simulink model "c00026M_harness"  (R2018a)
settings: Solver=ode3  StartTime=0.0  StopTime=10.0  RelTol=1e-3  EnableMultiTasking=on
undefined symbols (not defined in the file): b, DiscIntNeverNeededParam, J, K, L, PosMinimaW4, R, sigbuilder_block
(part 32 of 40)

== stateflow chart c00026M_harness/M008/Cyber/WL/Chart ==
  state Bajand_hasta_abajo
    entry: W = -1;
  state Bajando
    entry: W = -1;
  state Idle
    entry:W = 0;
  state Subiendo_hasta_arriba
    entry: W = 1;
  state Subiendo
    entry: W = 1;
  Subiendo -> Bajand_hasta_abajo [order 4] : [UI==4]
  Bajand_hasta_abajo -> Bajando [order 2] : [UI==3]
  Subiendo -> Bajando [order 3] : [UI==3]
  Bajando -> Bajand_hasta_abajo [order 2] : [UI==4]
  Idle -> Bajando [order 3] : [UI==3&&S>0]
  Subiendo_hasta_arriba -> Bajand_hasta_abajo [order 3] : [UI==4]
  Idle -> Bajand_hasta_abajo [order 4] : [UI==4&&S>0]
  Bajando -> Subiendo [order 3] : [UI==1]
  Subiendo_hasta_arriba -> Bajando [order 4] : [UI==3]
  Bajand_hasta_abajo -> Subiendo [order 4] : [UI==1]
  Bajand_hasta_abajo -> Idle [order 1] : [S<=0]
  Bajand_hasta_abajo -> Subiendo_hasta_arriba [order 3] : [UI==2]
  Bajando -> Idle [order 1] : [S<=0||UI==0]
  Bajando -> Subiendo_hasta_arriba [order 4] : [UI==2]
  (default) -> Idle
  Idle -> Subiendo_hasta_arriba [order 2] : [UI==2&&S<5]
  Idle -> Subiendo [order 1] : [UI == 1&&S<5]
  Subiendo -> Idle [order 1] : [S>=5||UI==0]
  Subiendo_hasta_arriba -> Idle [order 1] : [S >=5]
  Subiendo_hasta_arriba -> Subiendo [order 2] : [UI ==1]
  Subiendo -> Subiendo_hasta_arriba [order 2] : [UI==2]
  data: S input; UI input; W output double

== stateflow chart c00026M_harness/M008/Cyber/WL1/Chart1 ==
  state Bajand_hasta_abajo
    entry: W = -1;
  state Bajando
    entry: W = -1;
  state Idle
    entry:W = 0;
  state Subiendo_hasta_arriba
    entry: W = 1;
  state Subiendo
    entry: W = 1;
  Subiendo -> Bajand_hasta_abajo [order 4] : [UI==4]
  Bajand_hasta_abajo -> Bajando [order 2] : [UI==3]
  Subiendo -> Bajando [order 3] : [UI==3]
  Bajando -> Bajand_hasta_abajo [order 2] : [UI==4]
  Idle -> Bajando [order 3] : [UI==3&&S>0]
  Subiendo_hasta_arriba -> Bajand_hasta_abajo [order 3] : [UI==4]
  Idle -> Bajand_hasta_abajo [order 4] : [UI==4&&S>0]
  Bajando -> Subiendo [order 3] : [UI==1]
  Subiendo_hasta_arriba -> Bajando [order 4] : [UI==3]
  Bajand_hasta_abajo -> Subiendo [order 4] : [UI==1]
  Bajand_hasta_abajo -> Idle [order 1] : [S<=0]
  Bajand_hasta_abajo -> Subiendo_hasta_arriba [order 3] : [UI==2]
  Bajando -> Idle [order 1] : [S<=0||UI==0]
  Bajando -> Subiendo_hasta_arriba [order 4] : [UI==2]
  (default) -> Idle
  Idle -> Subiendo_hasta_arriba [order 2] : [UI==2&&S<5]
  Idle -> Subiendo [order 1] : [UI == 1&&S<5]
  Subiendo -> Idle [order 1] : [S>=5||UI==0]
  Subiendo_hasta_arriba -> Idle [order 1] : [S >=5]
  Subiendo_hasta_arriba -> Subiendo [order 2] : [UI ==1]
  Subiendo -> Subiendo_hasta_arriba [order 2] : [UI==2]
  data: S input; UI input; W output double

== stateflow chart c00026M_harness/M008/Cyber/WL3/Chart2 ==
  state Bajand_hasta_abajo
    entry: W = -1;
  state Bajando
    entry: W = -1;
  state Idle
    entry:W = 0;
  state Subiendo_hasta_arriba
    entry: W = 1;
  state Subiendo
    entry: W = 1;
  Subiendo -> Bajand_hasta_abajo [order 4] : [UI==4]
  Bajand_hasta_abajo -> Bajando [order 2] : [UI==3]
  Subiendo -> Bajando [order 3] : [UI==3]
  Bajando -> Bajand_hasta_abajo [order 2] : [UI==4]
  Idle -> Bajando [order 3] : [UI==3&&S>PosMinW4]
  Subiendo_hasta_arriba -> Bajand_hasta_abajo [order 3] : [UI==4]
  Idle -> Bajand_hasta_abajo [order 4] : [UI==4&&S>PosMinW4]
  Bajando -> Subiendo [order 3] : [UI==1]
  Subiendo_hasta_arriba -> Bajando [order 4] : [UI==3]
  Bajand_hasta_abajo -> Subiendo [order 4] : [UI==1]
  Bajand_hasta_abajo -> Idle [order 1] : [S<=PosMinW4]
  Bajand_hasta_abajo -> Subiendo_hasta_arriba [order 3] : [UI==2]
  Bajando -> Idle [order 1] : [S<=PosMinW4||UI==0]
  Bajando -> Subiendo_hasta_arriba [order 4] : [UI==2]
  (default) -> Idle
  Idle -> Subiendo_hasta_arriba [order 2] : [UI==2&&S<5]
  Idle -> Subiendo [order 1] : [UI == 1&&S<5]
  Subiendo -> Idle [order 1] : [S>=5||UI==0]
  Subiendo_hasta_arriba -> Idle [order 1] : [S >=5]
  Subiendo_hasta_arriba -> Subiendo [order 2] : [UI ==1]
  Subiendo -> Subiendo_hasta_arriba [order 2] : [UI==2]
  data: S input; UI input; W output double; PosMinW4 input

== stateflow chart c00026M_harness/M009/Cyber/WL/Chart ==
  state Bajand_hasta_abajo
    entry: W = -1;
  state Bajando
    entry: W = -1;
  state Idle
    entry:W = 0;
  state Subiendo_hasta_arriba
    entry: W = 1;
  state Subiendo
    entry: W = 1;
  Subiendo -> Bajand_hasta_abajo [order 4] : [UI==4]
  Bajand_hasta_abajo -> Bajando [order 2] : [UI==3]
  Subiendo -> Bajando [order 3] : [UI==3]
  Bajando -> Bajand_hasta_abajo [order 2] : [UI==4]
  Idle -> Bajando [order 3] : [UI==3&&S>0]
  Subiendo_hasta_arriba -> Bajand_hasta_abajo [order 3] : [UI==4]
  Idle -> Bajand_hasta_abajo [order 4] : [UI==4&&S>0]
  Bajando -> Subiendo [order 3] : [UI==1]
  Subiendo_hasta_arriba -> Bajando [order 4] : [UI==3]
  Bajand_hasta_abajo -> Subiendo [order 4] : [UI==1]
  Bajand_hasta_abajo -> Idle [order 1] : [S<=0]
  Bajand_hasta_abajo -> Subiendo_hasta_arriba [order 3] : [UI==2]
  Bajando -> Idle [order 1] : [S<=0||UI==0]
  Bajando -> Subiendo_hasta_arriba [order 4] : [UI==2]
  (default) -> Idle
  Idle -> Subiendo_hasta_arriba [order 2] : [UI==2&&S<5]
  Idle -> Subiendo [order 1] : [UI == 1&&S<5]
  Subiendo -> Idle [order 1] : [S>=5||UI==0]
  Subiendo_hasta_arriba -> Idle [order 1] : [S >=5]
  Subiendo_hasta_arriba -> Subiendo [order 2] : [UI ==1]
  Subiendo -> Subiendo_hasta_arriba [order 2] : [UI==2]
  data: S input; UI input; W output double

== stateflow chart c00026M_harness/M009/Cyber/WL1/Chart1 ==
  state Bajand_hasta_abajo
    entry: W = -1;
  state Bajando
    entry: W = -1;
  state Idle
    entry:W = 0;
  state Subiendo_hasta_arriba
    entry: W = 1;
  state Subiendo
    entry: W = 1;
  Subiendo -> Bajand_hasta_abajo [order 4] : [UI==4]
  Bajand_hasta_abajo -> Bajando [order 2] : [UI==3]
  Subiendo -> Bajando [order 3] : [UI==3]
  Bajando -> Bajand_hasta_abajo [order 2] : [UI==4]
  Idle -> Bajando [order 3] : [UI==3&&S>0]
  Subiendo_hasta_arriba -> Bajand_hasta_abajo [order 3] : [UI==4]
  Idle -> Bajand_hasta_abajo [order 4] : [UI==4&&S>0]
  Bajando -> Subiendo [order 3] : [UI==1]
  Subiendo_hasta_arriba -> Bajando [order 4] : [UI==3]
  Bajand_hasta_abajo -> Subiendo [order 4] : [UI==1]
  Bajand_hasta_abajo -> Idle [order 1] : [S<=0]
  Bajand_hasta_abajo -> Subiendo_hasta_arriba [order 3] : [UI==2]
  Bajando -> Idle [order 1] : [S<=0||UI==0]
  Bajando -> Subiendo_hasta_arriba [order 4] : [UI==2]
  (default) -> Idle
  Idle -> Subiendo_hasta_arriba [order 2] : [UI==2&&S<5]
  Idle -> Subiendo [order 1] : [UI == 1&&S<5]
  Subiendo -> Idle [order 1] : [S>=5||UI==0]
  Subiendo_hasta_arriba -> Idle [order 1] : [S >=5]
  Subiendo_hasta_arriba -> Subiendo [order 2] : [UI ==1]
  Subiendo -> Subiendo_hasta_arriba [order 2] : [UI==2]
  data: S input; UI input; W output double

== stateflow chart c00026M_harness/M009/Cyber/WL3/Chart2 ==
  state Bajand_hasta_abajo
    entry: W = -1;
  state Bajando
    entry: W = -1;
  state Idle
    entry:W = 0;
  state Subiendo_hasta_arriba
    entry: W = 1;
  state Subiendo
    entry: W = 1;
  Subiendo -> Bajand_hasta_abajo [order 4] : [UI==4]
  Bajand_hasta_abajo -> Bajando [order 2] : [UI==3]
  Subiendo -> Bajando [order 3] : [UI==3]
  Bajando -> Bajand_hasta_abajo [order 2] : [UI==4]
  Idle -> Bajando [order 3] : [UI==3&&S>PosMinW4]
  Subiendo_hasta_arriba -> Bajand_hasta_abajo [order 3] : [UI==4]
  Idle -> Bajand_hasta_abajo [order 4] : [UI==4&&S>PosMinW4]
  Bajando -> Subiendo [order 3] : [UI==1]
  Subiendo_hasta_arriba -> Bajando [order 4] : [UI==3]
  Bajand_hasta_abajo -> Subiendo [order 4] : [UI==1]
  Bajand_hasta_abajo -> Idle [order 1] : [S<=PosMinW4]
  Bajand_hasta_abajo -> Subiendo_hasta_arriba [order 3] : [UI==2]
  Bajando -> Idle [order 1] : [S<=PosMinW4||UI==0]
  Bajando -> Subiendo_hasta_arriba [order 4] : [UI==2]
  (default) -> Idle
  Idle -> Subiendo_hasta_arriba [order 2] : [UI==2&&S<5]
  Idle -> Subiendo [order 1] : [UI == 1&&S<5]
  Subiendo -> Idle [order 1] : [S>=5||UI==0]
  Subiendo_hasta_arriba -> Idle [order 1] : [S >=5]
  Subiendo_hasta_arriba -> Subiendo [order 2] : [UI ==1]
  Subiendo -> Subiendo_hasta_arriba [order 2] : [UI==2]
  data: S input; UI input; W output double; PosMinW4 input

== stateflow chart c00026M_harness/M010/Cyber/WL/Chart ==
  state Bajand_hasta_abajo
    entry: W = -1;
  state Bajando
    entry: W = -1;
  state Idle
    entry:W = 0;
  state Subiendo_hasta_arriba
    entry: W = 1;
  state Subiendo
    entry: W = 1;
  Subiendo -> Bajand_hasta_abajo [order 4] : [UI==4]
  Bajand_hasta_abajo -> Bajando [order 2] : [UI==3]
  Subiendo -> Bajando [order 3] : [UI==3]
  Bajando -> Bajand_hasta_abajo [order 2] : [UI==4]
  Idle -> Bajando [order 3] : [UI==3&&S>0]
  Subiendo_hasta_arriba -> Bajand_hasta_abajo [order 3] : [UI==4]
  Idle -> Bajand_hasta_abajo [order 4] : [UI==4&&S>0]
  Bajando -> Subiendo [order 3] : [UI==1]
  Subiendo_hasta_arriba -> Bajando [order 4] : [UI==3]
  Bajand_hasta_abajo -> Subiendo [order 4] : [UI==1]
  Bajand_hasta_abajo -> Idle [order 1] : [S<=0]
  Bajand_hasta_abajo -> Subiendo_hasta_arriba [order 3] : [UI==2]
  Bajando -> Idle [order 1] : [S<=0||UI==0]
  Bajando -> Subiendo_hasta_arriba [order 4] : [UI==2]
  (default) -> Idle
  Idle -> Subiendo_hasta_arriba [order 2] : [UI==2&&S<5]
  Idle -> Subiendo [order 1] : [UI == 1&&S<5]
  Subiendo -> Idle [order 1] : [S>=5||UI==0]
  Subiendo_hasta_arriba -> Idle [order 1] : [S >=5]
  Subiendo_hasta_arriba -> Subiendo [order 2] : [UI ==1]
  Subiendo -> Subiendo_hasta_arriba [order 2] : [UI==2]
  data: S input; UI input; W output double

== stateflow chart c00026M_harness/M010/Cyber/WL1/Chart1 ==
  state Bajand_hasta_abajo
    entry: W = -1;
  state Bajando
    entry: W = -1;
  state Idle
    entry:W = 0;
  state Subiendo_hasta_arriba
    entry: W = 1;
  state Subiendo
    entry: W = 1;
  Subiendo -> Bajand_hasta_abajo [order 4] : [UI==4]
  Bajand_hasta_abajo -> Bajando [order 2] : [UI==3]
  Subiendo -> Bajando [order 3] : [UI==3]
  Bajando -> Bajand_hasta_abajo [order 2] : [UI==4]
  Idle -> Bajando [order 3] : [UI==3&&S>0]
  Subiendo_hasta_arriba -> Bajand_hasta_abajo [order 3] : [UI==4]
  Idle -> Bajand_hasta_abajo [order 4] : [UI==4&&S>0]
  Bajando -> Subiendo [order 3] : [UI==1]
  Subiendo_hasta_arriba -> Bajando [order 4] : [UI==3]
  Bajand_hasta_abajo -> Subiendo [order 4] : [UI==1]
  Bajand_hasta_abajo -> Idle [order 1] : [S<=0]
  Bajand_hasta_abajo -> Subiendo_hasta_arriba [order 3] : [UI==2]
  Bajando -> Idle [order 1] : [S<=0||UI==0]
  Bajando -> Subiendo_hasta_arriba [order 4] : [UI==2]
  (default) -> Idle
  Idle -> Subiendo_hasta_arriba [order 2] : [UI==2&&S<5]
  Idle -> Subiendo [order 1] : [UI == 1&&S<5]
  Subiendo -> Idle [order 1] : [S>=5||UI==0]
  Subiendo_hasta_arriba -> Idle [order 1] : [S >=5]
  Subiendo_hasta_arriba -> Subiendo [order 2] : [UI ==1]
  Subiendo -> Subiendo_hasta_arriba [order 2] : [UI==2]
  data: S input; UI input; W output double

== stateflow chart c00026M_harness/M010/Cyber/WL3/Chart2 ==
  state Bajand_hasta_abajo
    entry: W = -1;
  state Bajando
    entry: W = -1;
  state Idle
    entry:W = 0;
  state Subiendo_hasta_arriba
    entry: W = 1;
  state Subiendo
    entry: W = 1;
  Subiendo -> Bajand_hasta_abajo [order 4] : [UI==4]
  Bajand_hasta_abajo -> Bajando [order 2] : [UI==3]
  Subiendo -> Bajando [order 3] : [UI==3]
  Bajando -> Bajand_hasta_abajo [order 2] : [UI==4]
  Idle -> Bajando [order 3] : [UI==3&&S>PosMinW4]
  Subiendo_hasta_arriba -> Bajand_hasta_abajo [order 3] : [UI==4]
  Idle -> Bajand_hasta_abajo [order 4] : [UI==4&&S>PosMinW4]
  Bajando -> Subiendo [order 3] : [UI==1]
  Subiendo_hasta_arriba -> Bajando [order 4] : [UI==3]
  Bajand_hasta_abajo -> Subiendo [order 4] : [UI==1]
  Bajand_hasta_abajo -> Idle [order 1] : [S<=PosMinW4]
  Bajand_hasta_abajo -> Subiendo_hasta_arriba [order 3] : [UI==2]
  Bajando -> Idle [order 1] : [S<=PosMinW4||UI==0]
  Bajando -> Subiendo_hasta_arriba [order 4] : [UI==2]
  (default) -> Idle
  Idle -> Subiendo_hasta_arriba [order 2] : [UI==2&&S<5]
  Idle -> Subiendo [order 1] : [UI == 1&&S<5]
  Subiendo -> Idle [order 1] : [S>=5||UI==0]
  Subiendo_hasta_arriba -> Idle [order 1] : [S >=5]
  Subiendo_hasta_arriba -> Subiendo [order 2] : [UI ==1]
  Subiendo -> Subiendo_hasta_arriba [order 2] : [UI==2]
  data: S input; UI input; W output double; PosMinW4 input

== stateflow chart c00026M_harness/M011/Cyber/WL/Chart ==
  state Bajand_hasta_abajo
    entry: W = -1;
  state Bajando
    entry: W = -1;
  state Idle
    entry:W = 0;
  state Subiendo_hasta_arriba
    entry: W = 1;
  state Subiendo
    entry: W = 1;
  Subiendo -> Bajand_hasta_abajo [order 4] : [UI==4]
  Bajand_hasta_abajo -> Bajando [order 2] : [UI==3]
  Subiendo -> Bajando [order 3] : [UI==3]
  Bajando -> Bajand_hasta_abajo [order 2] : [UI==4]
  Idle -> Bajando [order 3] : [UI==3&&S>0]
  Subiendo_hasta_arriba -> Bajand_hasta_abajo [order 3] : [UI==4]
  Idle -> Bajand_hasta_abajo [order 4] : [UI==4&&S>0]
  Bajando -> Subiendo [order 3] : [UI==1]
  Subiendo_hasta_arriba -> Bajando [order 4] : [UI==3]
  Bajand_hasta_abajo -> Subiendo [order 4] : [UI==1]
  Bajand_hasta_abajo -> Idle [order 1] : [S<=0]
  Bajand_hasta_abajo -> Subiendo_hasta_arriba [order 3] : [UI==2]
  Bajando -> Idle [order 1] : [S<=0||UI==0]
  Bajando -> Subiendo_hasta_arriba [order 4] : [UI==2]
  (default) -> Idle
  Idle -> Subiendo_hasta_arriba [order 2] : [UI==2&&S<5]
  Idle -> Subiendo [order 1] : [UI == 1&&S<5]
  Subiendo -> Idle [order 1] : [S>=5||UI==0]
  Subiendo_hasta_arriba -> Idle [order 1] : [S >=5]
  Subiendo_hasta_arriba -> Subiendo [order 2] : [UI ==1]
  Subiendo -> Subiendo_hasta_arriba [order 2] : [UI==2]
  data: S input; UI input; W output double

== stateflow chart c00026M_harness/M011/Cyber/WL1/Chart1 ==
  state Bajand_hasta_abajo
    entry: W = -1;
  state Bajando
    entry: W = -1;
  state Idle
    entry:W = 0;
  state Subiendo_hasta_arriba
    entry: W = 1;
  state Subiendo
    entry: W = 1;
  Subiendo -> Bajand_hasta_abajo [order 4] : [UI==4]
  Bajand_hasta_abajo -> Bajando [order 2] : [UI==3]
  Subiendo -> Bajando [order 3] : [UI==3]
  Bajando -> Bajand_hasta_abajo [order 2] : [UI==4]
  Idle -> Bajando [order 3] : [UI==3&&S>0]
  Subiendo_hasta_arriba -> Bajand_hasta_abajo [order 3] : [UI==4]
  Idle -> Bajand_hasta_abajo [order 4] : [UI==4&&S>0]
  Bajando -> Subiendo [order 3] : [UI==1]
  Subiendo_hasta_arriba -> Bajando [order 4] : [UI==3]
  Bajand_hasta_abajo -> Subiendo [order 4] : [UI==1]
  Bajand_hasta_abajo -> Idle [order 1] : [S<=0]
  Bajand_hasta_abajo -> Subiendo_hasta_arriba [order 3] : [UI==2]
  Bajando -> Idle [order 1] : [S<=0||UI==0]
  Bajando -> Subiendo_hasta_arriba [order 4] : [UI==2]
  (default) -> Idle
  Idle -> Subiendo_hasta_arriba [order 2] : [UI==2&&S<5]
  Idle -> Subiendo [order 1] : [UI == 1&&S<5]
  Subiendo -> Idle [order 1] : [S>=5||UI==0]
  Subiendo_hasta_arriba -> Idle [order 1] : [S >=5]
  Subiendo_hasta_arriba -> Subiendo [order 2] : [UI ==1]
  Subiendo -> Subiendo_hasta_arriba [order 2] : [UI==2]
  data: S input; UI input; W output double

== stateflow chart c00026M_harness/M011/Cyber/WL3/Chart2 ==
  state Bajand_hasta_abajo
    entry: W = -1;
  state Bajando
    entry: W = -1;
  state Idle
    entry:W = 0;
  state Subiendo_hasta_arriba
    entry: W = 1;
  state Subiendo
    entry: W = 1;
  Subiendo -> Bajand_hasta_abajo [order 4] : [UI==4]
  Bajand_hasta_abajo -> Bajando [order 2] : [UI==3]
  Subiendo -> Bajando [order 3] : [UI==3]
  Bajando -> Bajand_hasta_abajo [order 2] : [UI==4]
  Idle -> Bajando [order 3] : [UI==3&&S>PosMinW4]
  Subiendo_hasta_arriba -> Bajand_hasta_abajo [order 3] : [UI==4]
  Idle -> Bajand_hasta_abajo [order 4] : [UI==4&&S>PosMinW4]
  Bajando -> Subiendo [order 3] : [UI==1]
  Subiendo_hasta_arriba -> Bajando [order 4] : [UI==3]
  Bajand_hasta_abajo -> Subiendo [order 4] : [UI==1]
  Bajand_hasta_abajo -> Idle [order 1] : [S<=PosMinW4]
  Bajand_hasta_abajo -> Subiendo_hasta_arriba [order 3] : [UI==2]
  Bajando -> Idle [order 1] : [S<=PosMinW4||UI==0]
  Bajando -> Subiendo_hasta_arriba [order 4] : [UI==2]
  (default) -> Idle
  Idle -> Subiendo_hasta_arriba [order 2] : [UI==2&&S<5]
  Idle -> Subiendo [order 1] : [UI == 1&&S<5]
  Subiendo -> Idle [order 1] : [S>=5||UI==0]
  Subiendo_hasta_arriba -> Idle [order 1] : [S >=5]
  Subiendo_hasta_arriba -> Subiendo [order 2] : [UI ==1]
  Subiendo -> Subiendo_hasta_arriba [order 2] : [UI==2]
  data: S input; UI input; W output double; PosMinW4 input

== stateflow chart c00026M_harness/M012/Cyber/WL/Chart ==
  state Bajand_hasta_abajo
    entry: W = -1;
  state Bajando
    entry: W = -1;
  state Idle
    entry:W = 0;
  state Subiendo_hasta_arriba
    entry: W = 1;
  state Subiendo
    entry: W = 1;
  Subiendo -> Bajand_hasta_abajo [order 4] : [UI==4]
  Bajand_hasta_abajo -> Bajando [order 2] : [UI==3]
  Subiendo -> Bajando [order 3] : [UI==3]
  Bajando -> Bajand_hasta_abajo [order 2] : [UI==4]
  Idle -> Bajando [order 3] : [UI==3&&S>0]
  Subiendo_hasta_arriba -> Bajand_hasta_abajo [order 3] : [UI==4]
  Idle -> Bajand_hasta_abajo [order 4] : [UI==4&&S>0]
  Bajando -> Subiendo [order 3] : [UI==1]
  Subiendo_hasta_arriba -> Bajando [order 4] : [UI==3]
  Bajand_hasta_abajo -> Subiendo [order 4] : [UI==1]
  Bajand_hasta_abajo -> Idle [order 1] : [S<=0]
  Bajand_hasta_abajo -> Subiendo_hasta_arriba [order 3] : [UI==2]
  Bajando -> Idle [order 1] : [S<=0||UI==0]
  Bajando -> Subiendo_hasta_arriba [order 4] : [UI==2]
  (default) -> Idle
  Idle -> Subiendo_hasta_arriba [order 2] : [UI==2&&S<5]
  Idle -> Subiendo [order 1] : [UI == 1&&S<5]
  Subiendo -> Idle [order 1] : [S>=5||UI==0]
  Subiendo_hasta_arriba -> Idle [order 1] : [S >=5]
  Subiendo_hasta_arriba -> Subiendo [order 2] : [UI ==1]
  Subiendo -> Subiendo_hasta_arriba [order 2] : [UI==2]
  data: S input; UI input; W output double

== stateflow chart c00026M_harness/M012/Cyber/WL1/Chart1 ==
  state Bajand_hasta_abajo
    entry: W = -1;
  state Bajando
    entry: W = -1;
  state Idle
    entry:W = 0;
  state Subiendo_hasta_arriba
    entry: W = 1;
  state Subiendo
    entry: W = 1;
  Subiendo -> Bajand_hasta_abajo [order 4] : [UI==4]
  Bajand_hasta_abajo -> Bajando [order 2] : [UI==3]
  Subiendo -> Bajando [order 3] : [UI==3]
  Bajando -> Bajand_hasta_abajo [order 2] : [UI==4]
  Idle -> Bajando [order 3] : [UI==3&&S>0]
  Subiendo_hasta_arriba -> Bajand_hasta_abajo [order 3] : [UI==4]
  Idle -> Bajand_hasta_abajo [order 4] : [UI==4&&S>0]
  Bajando -> Subiendo [order 3] : [UI==1]
  Subiendo_hasta_arriba -> Bajando [order 4] : [UI==3]
  Bajand_hasta_abajo -> Subiendo [order 4] : [UI==1]
  Bajand_hasta_abajo -> Idle [order 1] : [S<=0]
  Bajand_hasta_abajo -> Subiendo_hasta_arriba [order 3] : [UI==2]
  Bajando -> Idle [order 1] : [S<=0||UI==0]
  Bajando -> Subiendo_hasta_arriba [order 4] : [UI==2]
  (default) -> Idle
  Idle -> Subiendo_hasta_arriba [order 2] : [UI==2&&S<5]
  Idle -> Subiendo [order 1] : [UI == 1&&S<5]
  Subiendo -> Idle [order 1] : [S>=5||UI==0]
  Subiendo_hasta_arriba -> Idle [order 1] : [S >=5]
  Subiendo_hasta_arriba -> Subiendo [order 2] : [UI ==1]
  Subiendo -> Subiendo_hasta_arriba [order 2] : [UI==2]
  data: S input; UI input; W output double

== stateflow chart c00026M_harness/M012/Cyber/WL3/Chart2 ==
  state Bajand_hasta_abajo
    entry: W = -1;
  state Bajando
    entry: W = -1;
  state Idle
    entry:W = 0;
  state Subiendo_hasta_arriba
    entry: W = 1;
  state Subiendo
    entry: W = 1;
  Subiendo -> Bajand_hasta_abajo [order 4] : [UI==4]
  Bajand_hasta_abajo -> Bajando [order 2] : [UI==3]
  Subiendo -> Bajando [order 3] : [UI==3]
  Bajando -> Bajand_hasta_abajo [order 2] : [UI==4]
  Idle -> Bajando [order 3] : [UI==3&&S>PosMinW4]
  Subiendo_hasta_arriba -> Bajand_hasta_abajo [order 3] : [UI==4]
  Idle -> Bajand_hasta_abajo [order 4] : [UI==4&&S>PosMinW4]
  Bajando -> Subiendo [order 3] : [UI==1]
  Subiendo_hasta_arriba -> Bajando [order 4] : [UI==3]
  Bajand_hasta_abajo -> Subiendo [order 4] : [UI==1]
  Bajand_hasta_abajo -> Idle [order 1] : [S<=PosMinW4]
  Bajand_hasta_abajo -> Subiendo_hasta_arriba [order 3] : [UI==2]
  Bajando -> Idle [order 1] : [S<=PosMinW4||UI==0]
  Bajando -> Subiendo_hasta_arriba [order 4] : [UI==2]
  (default) -> Idle
  Idle -> Subiendo_hasta_arriba [order 2] : [UI==2&&S<5]
  Idle -> Subiendo [order 1] : [UI == 1&&S<5]
  Subiendo -> Idle [order 1] : [S>=5||UI==0]
  Subiendo_hasta_arriba -> Idle [order 1] : [S >=5]
  Subiendo_hasta_arriba -> Subiendo [order 2] : [UI ==1]
  Subiendo -> Subiendo_hasta_arriba [order 2] : [UI==2]
  data: S input; UI input; W output double; PosMinW4 input

== stateflow chart c00026M_harness/M014/Cyber/WL/Chart ==
  state Bajand_hasta_abajo
    entry: W = -1;
  state Bajando
    entry: W = -1;
  state Idle
    entry:W = 0;
  state Subiendo_hasta_arriba
    entry: W = 1;
  state Subiendo
    entry: W = 1;
  Subiendo -> Bajand_hasta_abajo [order 4] : [UI==4]
  Bajand_hasta_abajo -> Bajando [order 2] : [UI==3]
  Subiendo -> Bajando [order 3] : [UI==3]
  Bajando -> Bajand_hasta_abajo [order 2] : [UI==4]
  Idle -> Bajando [order 3] : [UI==3&&S>0]
  Subiendo_hasta_arriba -> Bajand_hasta_abajo [order 3] : [UI==4]
  Idle -> Bajand_hasta_abajo [order 4] : [UI==4&&S>0]
  Bajando -> Subiendo [order 3] : [UI==1]
  Subiendo_hasta_arriba -> Bajando [order 4] : [UI==3]
  Bajand_hasta_abajo -> Subiendo [order 4] : [UI==1]
  Bajand_hasta_abajo -> Idle [order 1] : [S<=0]
  Bajand_hasta_abajo -> Subiendo_hasta_arriba [order 3] : [UI==2]
  Bajando -> Idle [order 1] : [S<=0||UI==0]
  Bajando -> Subiendo_hasta_arriba [order 4] : [UI==2]
  (default) -> Idle
  Idle -> Subiendo_hasta_arriba [order 2] : [UI==2&&S<5]
  Idle -> Subiendo [order 1] : [UI == 1&&S<5]
  Subiendo -> Idle [order 1] : [S>=5||UI==0]
  Subiendo_hasta_arriba -> Idle [order 1] : [S >=5]
  Subiendo_hasta_arriba -> Subiendo [order 2] : [UI ==1]
  Subiendo -> Subiendo_hasta_arriba [order 2] : [UI==2]
  data: S input; UI input; W output double

== stateflow chart c00026M_harness/M014/Cyber/WL1/Chart1 ==
  state Bajand_hasta_abajo
    entry: W = -1;
  state Bajando
    entry: W = -1;
  state Idle
    entry:W = 0;
  state Subiendo_hasta_arriba
    entry: W = 1;
  state Subiendo
    entry: W = 1;
  Subiendo -> Bajand_hasta_abajo [order 4] : [UI==4]
  Bajand_hasta_abajo -> Bajando [order 2] : [UI==3]
  Subiendo -> Bajando [order 3] : [UI==3]
  Bajando -> Bajand_hasta_abajo [order 2] : [UI==4]
  Idle -> Bajando [order 3] : [UI==3&&S>0]
  Subiendo_hasta_arriba -> Bajand_hasta_abajo [order 3] : [UI==4]
  Idle -> Bajand_hasta_abajo [order 4] : [UI==4&&S>0]
  Bajando -> Subiendo [order 3] : [UI==1]
  Subiendo_hasta_arriba -> Bajando [order 4] : [UI==3]
  Bajand_hasta_abajo -> Subiendo [order 4] : [UI==1]
  Bajand_hasta_abajo -> Idle [order 1] : [S<=0]
  Bajand_hasta_abajo -> Subiendo_hasta_arriba [order 3] : [UI==2]
  Bajando -> Idle [order 1] : [S<=0||UI==0]
  Bajando -> Subiendo_hasta_arriba [order 4] : [UI==2]
  (default) -> Idle
  Idle -> Subiendo_hasta_arriba [order 2] : [UI==2&&S<5]
  Idle -> Subiendo [order 1] : [UI == 1&&S<5]
  Subiendo -> Idle [order 1] : [S>=5||UI==0]
  Subiendo_hasta_arriba -> Idle [order 1] : [S >=5]
  Subiendo_hasta_arriba -> Subiendo [order 2] : [UI ==1]
  Subiendo -> Subiendo_hasta_arriba [order 2] : [UI==2]
  data: S input; UI input; W output double

== stateflow chart c00026M_harness/M014/Cyber/WL3/Chart2 ==
  state Bajand_hasta_abajo
    entry: W = -1;
  state Bajando
    entry: W = -1;
  state Idle
    entry:W = 0;
  state Subiendo_hasta_arriba
    entry: W = 1;
  state Subiendo
    entry: W = 1;
  Subiendo -> Bajand_hasta_abajo [order 4] : [UI==4]
  Bajand_hasta_abajo -> Bajando [order 2] : [UI==3]
  Subiendo -> Bajando [order 3] : [UI==3]
  Bajando -> Bajand_hasta_abajo [order 2] : [UI==4]
  Idle -> Bajando [order 3] : [UI==3&&S>PosMinW4]
  Subiendo_hasta_arriba -> Bajand_hasta_abajo [order 3] : [UI==4]
  Idle -> Bajand_hasta_abajo [order 4] : [UI==4&&S>PosMinW4]
  Bajando -> Subiendo [order 3] : [UI==1]
  Subiendo_hasta_arriba -> Bajando [order 4] : [UI==3]
  Bajand_hasta_abajo -> Subiendo [order 4] : [UI==1]
  Bajand_hasta_abajo -> Idle [order 1] : [S<=PosMinW4]
  Bajand_hasta_abajo -> Subiendo_hasta_arriba [order 3] : [UI==2]
  Bajando -> Idle [order 1] : [S<=PosMinW4||UI==0]
  Bajando -> Subiendo_hasta_arriba [order 4] : [UI==2]
  (default) -> Idle
  Idle -> Subiendo_hasta_arriba [order 2] : [UI==2&&S<5]
  Idle -> Subiendo [order 1] : [UI == 1&&S<5]
  Subiendo -> Idle [order 1] : [S>=5||UI==0]
  Subiendo_hasta_arriba -> Idle [order 1] : [S >=5]
  Subiendo_hasta_arriba -> Subiendo [order 2] : [UI ==1]
  Subiendo -> Subiendo_hasta_arriba [order 2] : [UI==2]
  data: S input; UI input; W output double; PosMinW4 input

== stateflow chart c00026M_harness/M015/Cyber/WL/Chart ==
  state Bajand_hasta_abajo
    entry: W = -1;
  state Bajando
    entry: W = 0;
  state Idle
    entry:W = 0;
  state Subiendo_hasta_arriba
    entry: W = 1;
  state Subiendo
    entry: W = 1;
  Subiendo -> Bajand_hasta_abajo [order 4] : [UI==4]
  Bajand_hasta_abajo -> Bajando [order 2] : [UI==3]
  Subiendo -> Bajando [order 3] : [UI==3]
  Bajando -> Bajand_hasta_abajo [order 2] : [UI==4]
  Idle -> Bajando [order 3] : [UI==3&&S>0]
  Subiendo_hasta_arriba -> Bajand_hasta_abajo [order 3] : [UI==4]
  Idle -> Bajand_hasta_abajo [order 4] : [UI==4&&S>0]
  Bajando -> Subiendo [order 3] : [UI==1]
  Subiendo_hasta_arriba -> Bajando [order 4] : [UI==3]
  Bajand_hasta_abajo -> Subiendo [order 4] : [UI==1]
  Bajand_hasta_abajo -> Idle [order 1] : [S<=0]
  Bajand_hasta_abajo -> Subiendo_hasta_arriba [order 3] : [UI==2]
  Bajando -> Idle [order 1] : [S<=0||UI==0]
  Bajando -> Subiendo_hasta_arriba [order 4] : [UI==2]
  (default) -> Idle
  Idle -> Subiendo_hasta_arriba [order 2] : [UI==2&&S<5]
  Idle -> Subiendo [order 1] : [UI == 1&&S<5]
  Subiendo -> Idle [order 1] : [S>=5||UI==0]
  Subiendo_hasta_arriba -> Idle [order 1] : [S >=5]
  Subiendo_hasta_arriba -> Subiendo [order 2] : [UI ==1]
  Subiendo -> Subiendo_hasta_arriba [order 2] : [UI==2]
  data: S input; UI input; W output double

== stateflow chart c00026M_harness/M015/Cyber/WL1/Chart1 ==
  state Bajand_hasta_abajo
    entry: W = -1;
  state Bajando
    entry: W = -1;
  state Idle
    entry:W = 0;
  state Subiendo_hasta_arriba
    entry: W = 1;
  state Subiendo
    entry: W = 1;
  Subiendo -> Bajand_hasta_abajo [order 4] : [UI==4]
  Bajand_hasta_abajo -> Bajando [order 2] : [UI==3]
  Subiendo -> Bajando [order 3] : [UI==3]
  Bajando -> Bajand_hasta_abajo [order 2] : [UI==4]
  Idle -> Bajando [order 3] : [UI==3&&S>0]
  Subiendo_hasta_arriba -> Bajand_hasta_abajo [order 3] : [UI==4]
  Idle -> Bajand_hasta_abajo [order 4] : [UI==4&&S>0]
  Bajando -> Subiendo [order 3] : [UI==1]
  Subiendo_hasta_arriba -> Bajando [order 4] : [UI==3]
  Bajand_hasta_abajo -> Subiendo [order 4] : [UI==1]
  Bajand_hasta_abajo -> Idle [order 1] : [S<=0]
  Bajand_hasta_abajo -> Subiendo_hasta_arriba [order 3] : [UI==2]
  Bajando -> Idle [order 1] : [S<=0||UI==0]
  Bajando -> Subiendo_hasta_arriba [order 4] : [UI==2]
  (default) -> Idle
  Idle -> Subiendo_hasta_arriba [order 2] : [UI==2&&S<5]
  Idle -> Subiendo [order 1] : [UI == 1&&S<5]
  Subiendo -> Idle [order 1] : [S>=5||UI==0]
  Subiendo_hasta_arriba -> Idle [order 1] : [S >=5]
  Subiendo_hasta_arriba -> Subiendo [order 2] : [UI ==1]
  Subiendo -> Subiendo_hasta_arriba [order 2] : [UI==2]
  data: S input; UI input; W output double

== stateflow chart c00026M_harness/M015/Cyber/WL3/Chart2 ==
  state Bajand_hasta_abajo
    entry: W = -1;
  state Bajando
    entry: W = -1;
  state Idle
    entry:W = 0;
  state Subiendo_hasta_arriba
    entry: W = 1;
  state Subiendo
    entry: W = 1;
  Subiendo -> Bajand_hasta_abajo [order 4] : [UI==4]
  Bajand_hasta_abajo -> Bajando [order 2] : [UI==3]
  Subiendo -> Bajando [order 3] : [UI==3]
  Bajando -> Bajand_hasta_abajo [order 2] : [UI==4]
  Idle -> Bajando [order 3] : [UI==3&&S>PosMinW4]
  Subiendo_hasta_arriba -> Bajand_hasta_abajo [order 3] : [UI==4]
  Idle -> Bajand_hasta_abajo [order 4] : [UI==4&&S>PosMinW4]
  Bajando -> Subiendo [order 3] : [UI==1]
  Subiendo_hasta_arriba -> Bajando [order 4] : [UI==3]
  Bajand_hasta_abajo -> Subiendo [order 4] : [UI==1]
  Bajand_hasta_abajo -> Idle [order 1] : [S<=PosMinW4]
  Bajand_hasta_abajo -> Subiendo_hasta_arriba [order 3] : [UI==2]
  Bajando -> Idle [order 1] : [S<=PosMinW4||UI==0]
  Bajando -> Subiendo_hasta_arriba [order 4] : [UI==2]
  (default) -> Idle
  Idle -> Subiendo_hasta_arriba [order 2] : [UI==2&&S<5]
  Idle -> Subiendo [order 1] : [UI == 1&&S<5]
  Subiendo -> Idle [order 1] : [S>=5||UI==0]
  Subiendo_hasta_arriba -> Idle [order 1] : [S >=5]
  Subiendo_hasta_arriba -> Subiendo [order 2] : [UI ==1]
  Subiendo -> Subiendo_hasta_arriba [order 2] : [UI==2]
  data: S input; UI input; W output double; PosMinW4 input

== stateflow chart c00026M_harness/M016/Cyber/WL/Chart ==
  state Bajand_hasta_abajo
    entry: W = -1;
  state Bajando
    entry: W = -1;
  state Idle
    entry:W = 0;
  state Subiendo_hasta_arriba
    entry: W = 1;
  state Subiendo
    entry: W = 1;
  Subiendo -> Bajand_hasta_abajo [order 4] : [UI==4]
  Bajand_hasta_abajo -> Bajando [order 2] : [UI==3]
  Subiendo -> Bajando [order 3] : [UI==3]
  Bajando -> Bajand_hasta_abajo [order 2] : [UI==4]
  Idle -> Bajando [order 3] : [UI==3&&S>0]
  Subiendo_hasta_arriba -> Bajand_hasta_abajo [order 3] : [UI==4]
  Idle -> Bajand_hasta_abajo [order 4] : [UI==4&&S>0]
  Bajando -> Subiendo [order 3] : [UI==1]
  Subiendo_hasta_arriba -> Bajando [order 4] : [UI==3]
  Bajand_hasta_abajo -> Subiendo [order 4] : [UI==1]
  Bajand_hasta_abajo -> Idle [order 1] : [S<=0]
  Bajand_hasta_abajo -> Subiendo_hasta_arriba [order 3] : [UI==2]
  Bajando -> Idle [order 1] : [S<=0||UI==0]
  Bajando -> Subiendo_hasta_arriba [order 4] : [UI==2]
  (default) -> Idle
  Idle -> Subiendo_hasta_arriba [order 2] : [UI==2&&S<5]
  Idle -> Subiendo [order 1] : [UI == 1&&S<5]
  Subiendo -> Idle [order 1] : [S>=5||UI==0]
  Subiendo_hasta_arriba -> Idle [order 1] : [S >=5]
  Subiendo_hasta_arriba -> Subiendo [order 2] : [UI ==1]
  Subiendo -> Subiendo_hasta_arriba [order 2] : [UI==2]
  data: S input; UI input; W output double

== stateflow chart c00026M_harness/M016/Cyber/WL1/Chart1 ==
  state Bajand_hasta_abajo
    entry: W = -1;
  state Bajando
    entry: W = 0;
  state Idle
    entry:W = 0;
  state Subiendo_hasta_arriba
    entry: W = 1;
  state Subiendo
    entry: W = 1;
  Subiendo -> Bajand_hasta_abajo [order 4] : [UI==4]
  Bajand_hasta_abajo -> Bajando [order 2] : [UI==3]
  Subiendo -> Bajando [order 3] : [UI==3]
  Bajando -> Bajand_hasta_abajo [order 2] : [UI==4]
  Idle -> Bajando [order 3] : [UI==3&&S>0]
  Subiendo_hasta_arriba -> Bajand_hasta_abajo [order 3] : [UI==4]
  Idle -> Bajand_hasta_abajo [order 4] : [UI==4&&S>0]
  Bajando -> Subiendo [order 3] : [UI==1]
  Subiendo_hasta_arriba -> Bajando [order 4] : [UI==3]
  Bajand_hasta_abajo -> Subiendo [order 4] : [UI==1]
  Bajand_hasta_abajo -> Idle [order 1] : [S<=0]
  Bajand_hasta_abajo -> Subiendo_hasta_arriba [order 3] : [UI==2]
  Bajando -> Idle [order 1] : [S<=0||UI==0]
  Bajando -> Subiendo_hasta_arriba [order 4] : [UI==2]
  (default) -> Idle
  Idle -> Subiendo_hasta_arriba [order 2] : [UI==2&&S<5]
  Idle -> Subiendo [order 1] : [UI == 1&&S<5]
  Subiendo -> Idle [order 1] : [S>=5||UI==0]
  Subiendo_hasta_arriba -> Idle [order 1] : [S >=5]
  Subiendo_hasta_arriba -> Subiendo [order 2] : [UI ==1]
  Subiendo -> Subiendo_hasta_arriba [order 2] : [UI==2]
  data: S input; UI input; W output double

== stateflow chart c00026M_harness/M016/Cyber/WL3/Chart2 ==
  state Bajand_hasta_abajo
    entry: W = -1;
  state Bajando
    entry: W = -1;
  state Idle
    entry:W = 0;
  state Subiendo_hasta_arriba
    entry: W = 1;
  state Subiendo
    entry: W = 1;
  Subiendo -> Bajand_hasta_abajo [order 4] : [UI==4]
  Bajand_hasta_abajo -> Bajando [order 2] : [UI==3]
  Subiendo -> Bajando [order 3] : [UI==3]
  Bajando -> Bajand_hasta_abajo [order 2] : [UI==4]
  Idle -> Bajando [order 3] : [UI==3&&S>PosMinW4]
  Subiendo_hasta_arriba -> Bajand_hasta_abajo [order 3] : [UI==4]
  Idle -> Bajand_hasta_abajo [order 4] : [UI==4&&S>PosMinW4]
  Bajando -> Subiendo [order 3] : [UI==1]
  Subiendo_hasta_arriba -> Bajando [order 4] : [UI==3]
  Bajand_hasta_abajo -> Subiendo [order 4] : [UI==1]
  Bajand_hasta_abajo -> Idle [order 1] : [S<=PosMinW4]
  Bajand_hasta_abajo -> Subiendo_hasta_arriba [order 3] : [UI==2]
  Bajando -> Idle [order 1] : [S<=PosMinW4||UI==0]
  Bajando -> Subiendo_hasta_arriba [order 4] : [UI==2]
  (default) -> Idle
  Idle -> Subiendo_hasta_arriba [order 2] : [UI==2&&S<5]
  Idle -> Subiendo [order 1] : [UI == 1&&S<5]
  Subiendo -> Idle [order 1] : [S>=5||UI==0]
  Subiendo_hasta_arriba -> Idle [order 1] : [S >=5]
  Subiendo_hasta_arriba -> Subiendo [order 2] : [UI ==1]
  Subiendo -> Subiendo_hasta_arriba [order 2] : [UI==2]
  data: S input; UI input; W output double; PosMinW4 input

== stateflow chart c00026M_harness/M018/Cyber/WL/Chart ==
  state Bajand_hasta_abajo
    entry: W = -1;
  state Bajando
    entry: W = -1;
  state Idle
    entry:W = 0;
  state Subiendo_hasta_arriba
    entry: W = 1;
  state Subiendo
    entry: W = 1;
  Subiendo -> Bajand_hasta_abajo [order 4] : [UI==4]
  Bajand_hasta_abajo -> Bajando [order 2] : [UI==3]
  Subiendo -> Bajando [order 3] : [UI==3]
  Bajando -> Bajand_hasta_abajo [order 2] : [UI==4]
  Idle -> Bajando [order 3] : [UI==3&&S>0]
  Subiendo_hasta_arriba -> Bajand_hasta_abajo [order 3] : [UI==4]
  Idle -> Bajand_hasta_abajo [order 4] : [UI==4&&S>0]
  Bajando -> Subiendo [order 3] : [UI==1]
  Subiendo_hasta_arriba -> Bajando [order 4] : [UI==3]
  Bajand_hasta_abajo -> Subiendo [order 4] : [UI==1]
  Bajand_hasta_abajo -> Idle [order 1] : [S<=0]
  Bajand_hasta_abajo -> Subiendo_hasta_arriba [order 3] : [UI==2]
  Bajando -> Idle [order 1] : [S<=0||UI==0]
  Bajando -> Subiendo_hasta_arriba [order 4] : [UI==2]
  (default) -> Idle
  Idle -> Subiendo_hasta_arriba [order 2] : [UI==2&&S<5]
  Idle -> Subiendo [order 1] : [UI == 1&&S<5]
  Subiendo -> Idle [order 1] : [S>=5||UI==0]
  Subiendo_hasta_arriba -> Idle [order 1] : [S >=5]
  Subiendo_hasta_arriba -> Subiendo [order 2] : [UI ==1]
  Subiendo -> Subiendo_hasta_arriba [order 2] : [UI==2]
  data: S input; UI input; W output double

== stateflow chart c00026M_harness/M018/Cyber/WL1/Chart1 ==
  state Bajand_hasta_abajo
    entry: W = -1;
  state Bajando
    entry: W = -1;
  state Idle
    entry:W = 0;
  state Subiendo_hasta_arriba
    entry: W = 1;
  state Subiendo
    entry: W = 1;
  Subiendo -> Bajand_hasta_abajo [order 4] : [UI==4]
  Bajand_hasta_abajo -> Bajando [order 2] : [UI==3]
  Subiendo -> Bajando [order 3] : [UI==3]
  Bajando -> Bajand_hasta_abajo [order 2] : [UI==4]
  Idle -> Bajando [order 3] : [UI==3&&S>0]
  Subiendo_hasta_arriba -> Bajand_hasta_abajo [order 3] : [UI==4]
  Idle -> Bajand_hasta_abajo [order 4] : [UI==4&&S>0]
  Bajando -> Subiendo [order 3] : [UI==1]
  Subiendo_hasta_arriba -> Bajando [order 4] : [UI==3]
  Bajand_hasta_abajo -> Subiendo [order 4] : [UI==1]
  Bajand_hasta_abajo -> Idle [order 1] : [S<=0]
  Bajand_hasta_abajo -> Subiendo_hasta_arriba [order 3] : [UI==2]
  Bajando -> Idle [order 1] : [S<=0||UI==0]
  Bajando -> Subiendo_hasta_arriba [order 4] : [UI==2]
  (default) -> Idle
  Idle -> Subiendo_hasta_arriba [order 2] : [UI==2&&S<5]
  Idle -> Subiendo [order 1] : [UI == 1&&S<5]
  Subiendo -> Idle [order 1] : [S>=5||UI==0]
  Subiendo_hasta_arriba -> Idle [order 1] : [S >=5]
  Subiendo_hasta_arriba -> Subiendo [order 2] : [UI ==1]
  Subiendo -> Subiendo_hasta_arriba [order 2] : [UI==2]
  data: S input; UI input; W output double

== stateflow chart c00026M_harness/M018/Cyber/WL3/Chart2 ==
  state Bajand_hasta_abajo
    entry: W = -1;
  state Bajando
    entry: W = 0;
  state Idle
    entry:W = 0;
  state Subiendo_hasta_arriba
    entry: W = 1;
  state Subiendo
    entry: W = 1;
  Subiendo -> Bajand_hasta_abajo [order 4] : [UI==4]
  Bajand_hasta_abajo -> Bajando [order 2] : [UI==3]
  Subiendo -> Bajando [order 3] : [UI==3]
  Bajando -> Bajand_hasta_abajo [order 2] : [UI==4]
  Idle -> Bajando [order 3] : [UI==3&&S>PosMinW4]
  Subiendo_hasta_arriba -> Bajand_hasta_abajo [order 3] : [UI==4]
  Idle -> Bajand_hasta_abajo [order 4] : [UI==4&&S>PosMinW4]
  Bajando -> Subiendo [order 3] : [UI==1]
  Subiendo_hasta_arriba -> Bajando [order 4] : [UI==3]
  Bajand_hasta_abajo -> Subiendo [order 4] : [UI==1]
  Bajand_hasta_abajo -> Idle [order 1] : [S<=PosMinW4]
  Bajand_hasta_abajo -> Subiendo_hasta_arriba [order 3] : [UI==2]
  Bajando -> Idle [order 1] : [S<=PosMinW4||UI==0]
  Bajando -> Subiendo_hasta_arriba [order 4] : [UI==2]
  (default) -> Idle
  Idle -> Subiendo_hasta_arriba [order 2] : [UI==2&&S<5]
  Idle -> Subiendo [order 1] : [UI == 1&&S<5]
  Subiendo -> Idle [order 1] : [S>=5||UI==0]
  Subiendo_hasta_arriba -> Idle [order 1] : [S >=5]
  Subiendo_hasta_arriba -> Subiendo [order 2] : [UI ==1]
  Subiendo -> Subiendo_hasta_arriba [order 2] : [UI==2]
  data: S input; UI input; W output double; PosMinW4 input

== stateflow chart c00026M_harness/M019/Cyber/WL/Chart ==
  state Bajand_hasta_abajo
    entry: W = 0;
  state Bajando
    entry: W = -1;
  state Idle
    entry:W = 0;
  state Subiendo_hasta_arriba
    entry: W = 1;
  state Subiendo
    entry: W = 1;
  Subiendo -> Bajand_hasta_abajo [order 4] : [UI==4]
  Bajand_hasta_abajo -> Bajando [order 2] : [UI==3]
  Subiendo -> Bajando [order 3] : [UI==3]
  Bajando -> Bajand_hasta_abajo [order 2] : [UI==4]
  Idle -> Bajando [order 3] : [UI==3&&S>0]
  Subiendo_hasta_arriba -> Bajand_hasta_abajo [order 3] : [UI==4]
  Idle -> Bajand_hasta_abajo [order 4] : [UI==4&&S>0]
  Bajando -> Subiendo [order 3] : [UI==1]
  Subiendo_hasta_arriba -> Bajando [order 4] : [UI==3]
  Bajand_hasta_abajo -> Subiendo [order 4] : [UI==1]
  Bajand_hasta_abajo -> Idle [order 1] : [S<=0]
  Bajand_hasta_abajo -> Subiendo_hasta_arriba [order 3] : [UI==2]
  Bajando -> Idle [order 1] : [S<=0||UI==0]
  Bajando -> Subiendo_hasta_arriba [order 4] : [UI==2]
  (default) -> Idle
  Idle -> Subiendo_hasta_arriba [order 2] : [UI==2&&S<5]
  Idle -> Subiendo [order 1] : [UI == 1&&S<5]
  Subiendo -> Idle [order 1] : [S>=5||UI==0]
  Subiendo_hasta_arriba -> Idle [order 1] : [S >=5]
  Subiendo_hasta_arriba -> Subiendo [order 2] : [UI ==1]
  Subiendo -> Subiendo_hasta_arriba [order 2] : [UI==2]
  data: S input; UI input; W output double

== stateflow chart c00026M_harness/M019/Cyber/WL1/Chart1 ==
  state Bajand_hasta_abajo
    entry: W = -1;
  state Bajando
    entry: W = -1;
  state Idle
    entry:W = 0;
  state Subiendo_hasta_arriba
    entry: W = 1;
  state Subiendo
    entry: W = 1;
  Subiendo -> Bajand_hasta_abajo [order 4] : [UI==4]
  Bajand_hasta_abajo -> Bajando [order 2] : [UI==3]
  Subiendo -> Bajando [order 3] : [UI==3]
  Bajando -> Bajand_hasta_abajo [order 2] : [UI==4]
  Idle -> Bajando [order 3] : [UI==3&&S>0]
  Subiendo_hasta_arriba -> Bajand_hasta_abajo [order 3] : [UI==4]
  Idle -> Bajand_hasta_abajo [order 4] : [UI==4&&S>0]
  Bajando -> Subiendo [order 3] : [UI==1]
  Subiendo_hasta_arriba -> Bajando [order 4] : [UI==3]
  Bajand_hasta_abajo -> Subiendo [order 4] : [UI==1]
  Bajand_hasta_abajo -> Idle [order 1] : [S<=0]
  Bajand_hasta_abajo -> Subiendo_hasta_arriba [order 3] : [UI==2]
  Bajando -> Idle [order 1] : [S<=0||UI==0]
  Bajando -> Subiendo_hasta_arriba [order 4] : [UI==2]
  (default) -> Idle
  Idle -> Subiendo_hasta_arriba [order 2] : [UI==2&&S<5]
  Idle -> Subiendo [order 1] : [UI == 1&&S<5]
  Subiendo -> Idle [order 1] : [S>=5||UI==0]
  Subiendo_hasta_arriba -> Idle [order 1] : [S >=5]
  Subiendo_hasta_arriba -> Subiendo [order 2] : [UI ==1]
  Subiendo -> Subiendo_hasta_arriba [order 2] : [UI==2]
  data: S input; UI input; W output double

== stateflow chart c00026M_harness/M019/Cyber/WL3/Chart2 ==
  state Bajand_hasta_abajo
    entry: W = -1;
  state Bajando
    entry: W = -1;
  state Idle
    entry:W = 0;
  state Subiendo_hasta_arriba
    entry: W = 1;
  state Subiendo
    entry: W = 1;
  Subiendo -> Bajand_hasta_abajo [order 4] : [UI==4]
  Bajand_hasta_abajo -> Bajando [order 2] : [UI==3]
  Subiendo -> Bajando [order 3] : [UI==3]
  Bajando -> Bajand_hasta_abajo [order 2] : [UI==4]
  Idle -> Bajando [order 3] : [UI==3&&S>PosMinW4]
  Subiendo_hasta_arriba -> Bajand_hasta_abajo [order 3] : [UI==4]
  Idle -> Bajand_hasta_abajo [order 4] : [UI==4&&S>PosMinW4]
  Bajando -> Subiendo [order 3] : [UI==1]
  Subiendo_hasta_arriba -> Bajando [order 4] : [UI==3]
  Bajand_hasta_abajo -> Subiendo [order 4] : [UI==1]
  Bajand_hasta_abajo -> Idle [order 1] : [S<=PosMinW4]
  Bajand_hasta_abajo -> Subiendo_hasta_arriba [order 3] : [UI==2]
  Bajando -> Idle [order 1] : [S<=PosMinW4||UI==0]
  Bajando -> Subiendo_hasta_arriba [order 4] : [UI==2]
  (default) -> Idle
  Idle -> Subiendo_hasta_arriba [order 2] : [UI==2&&S<5]
  Idle -> Subiendo [order 1] : [UI == 1&&S<5]
  Subiendo -> Idle [order 1] : [S>=5||UI==0]
  Subiendo_hasta_arriba -> Idle [order 1] : [S >=5]
  Subiendo_hasta_arriba -> Subiendo [order 2] : [UI ==1]
  Subiendo -> Subiendo_hasta_arriba [order 2] : [UI==2]
  data: S input; UI input; W output double; PosMinW4 input

== stateflow chart c00026M_harness/M020/Cyber/WL/Chart ==
  state Bajand_hasta_abajo
    entry: W = -1;
  state Bajando
    entry: W = -1;
  state Idle
    entry:W = 0;
  state Subiendo_hasta_arriba
    entry: W = 1;
  state Subiendo
    entry: W = 1;
  Subiendo -> Bajand_hasta_abajo [order 4] : [UI==4]
  Bajand_hasta_abajo -> Bajando [order 2] : [UI==3]
  Subiendo -> Bajando [order 3] : [UI==3]
  Bajando -> Bajand_hasta_abajo [order 2] : [UI==4]
  Idle -> Bajando [order 3] : [UI==3&&S>0]
  Subiendo_hasta_arriba -> Bajand_hasta_abajo [order 3] : [UI==4]
  Idle -> Bajand_hasta_abajo [order 4] : [UI==4&&S>0]
  Bajando -> Subiendo [order 3] : [UI==1]
  Subiendo_hasta_arriba -> Bajando [order 4] : [UI==3]
  Bajand_hasta_abajo -> Subiendo [order 4] : [UI==1]
  Bajand_hasta_abajo -> Idle [order 1] : [S<=0]
  Bajand_hasta_abajo -> Subiendo_hasta_arriba [order 3] : [UI==2]
  Bajando -> Idle [order 1] : [S<=0||UI==0]
  Bajando -> Subiendo_hasta_arriba [order 4] : [UI==2]
  (default) -> Idle
  Idle -> Subiendo_hasta_arriba [order 2] : [UI==2&&S<5]
  Idle -> Subiendo [order 1] : [UI == 1&&S<5]
  Subiendo -> Idle [order 1] : [S>=5||UI==0]
  Subiendo_hasta_arriba -> Idle [order 1] : [S >=5]
  Subiendo_hasta_arriba -> Subiendo [order 2] : [UI ==1]
  Subiendo -> Subiendo_hasta_arriba [order 2] : [UI==2]
  data: S input; UI input; W output double

== stateflow chart c00026M_harness/M020/Cyber/WL1/Chart1 ==
  state Bajand_hasta_abajo
    entry: W = 0;
  state Bajando
    entry: W = -1;
  state Idle
    entry:W = 0;
  state Subiendo_hasta_arriba
    entry: W = 1;
  state Subiendo
    entry: W = 1;
  Subiendo -> Bajand_hasta_abajo [order 4] : [UI==4]
  Bajand_hasta_abajo -> Bajando [order 2] : [UI==3]
  Subiendo -> Bajando [order 3] : [UI==3]
  Bajando -> Bajand_hasta_abajo [order 2] : [UI==4]
  Idle -> Bajando [order 3] : [UI==3&&S>0]
  Subiendo_hasta_arriba -> Bajand_hasta_abajo [order 3] : [UI==4]
  Idle -> Bajand_hasta_abajo [order 4] : [UI==4&&S>0]
  Bajando -> Subiendo [order 3] : [UI==1]
  Subiendo_hasta_arriba -> Bajando [order 4] : [UI==3]
  Bajand_hasta_abajo -> Subiendo [order 4] : [UI==1]
  Bajand_hasta_abajo -> Idle [order 1] : [S<=0]
  Bajand_hasta_abajo -> Subiendo_hasta_arriba [order 3] : [UI==2]
  Bajando -> Idle [order 1] : [S<=0||UI==0]
  Bajando -> Subiendo_hasta_arriba [order 4] : [UI==2]
  (default) -> Idle
  Idle -> Subiendo_hasta_arriba [order 2] : [UI==2&&S<5]
  Idle -> Subiendo [order 1] : [UI == 1&&S<5]
  Subiendo -> Idle [order 1] : [S>=5||UI==0]
  Subiendo_hasta_arriba -> Idle [order 1] : [S >=5]
  Subiendo_hasta_arriba -> Subiendo [order 2] : [UI ==1]
  Subiendo -> Subiendo_hasta_arriba [order 2] : [UI==2]
  data: S input; UI input; W output double

== stateflow chart c00026M_harness/M020/Cyber/WL3/Chart2 ==
  state Bajand_hasta_abajo
    entry: W = -1;
  state Bajando
    entry: W = -1;
  state Idle
    entry:W = 0;
  state Subiendo_hasta_arriba
    entry: W = 1;
  state Subiendo
    entry: W = 1;
  Subiendo -> Bajand_hasta_abajo [order 4] : [UI==4]
  Bajand_hasta_abajo -> Bajando [order 2] : [UI==3]
  Subiendo -> Bajando [order 3] : [UI==3]
  Bajando -> Bajand_hasta_abajo [order 2] : [UI==4]
  Idle -> Bajando [order 3] : [UI==3&&S>PosMinW4]
  Subiendo_hasta_arriba -> Bajand_hasta_abajo [order 3] : [UI==4]
  Idle -> Bajand_hasta_abajo [order 4] : [UI==4&&S>PosMinW4]
  Bajando -> Subiendo [order 3] : [UI==1]
  Subiendo_hasta_arriba -> Bajando [order 4] : [UI==3]
  Bajand_hasta_abajo -> Subiendo [order 4] : [UI==1]
  Bajand_hasta_abajo -> Idle [order 1] : [S<=PosMinW4]
  Bajand_hasta_abajo -> Subiendo_hasta_arriba [order 3] : [UI==2]
  Bajando -> Idle [order 1] : [S<=PosMinW4||UI==0]
  Bajando -> Subiendo_hasta_arriba [order 4] : [UI==2]
  (default) -> Idle
  Idle -> Subiendo_hasta_arriba [order 2] : [UI==2&&S<5]
  Idle -> Subiendo [order 1] : [UI == 1&&S<5]
  Subiendo -> Idle [order 1] : [S>=5||UI==0]
  Subiendo_hasta_arriba -> Idle [order 1] : [S >=5]
  Subiendo_hasta_arriba -> Subiendo [order 2] : [UI ==1]
  Subiendo -> Subiendo_hasta_arriba [order 2] : [UI==2]
  data: S input; UI input; W output double; PosMinW4 input

== stateflow chart c00026M_harness/M022/Cyber/WL/Chart ==
  state Bajand_hasta_abajo
    entry: W = -1;
  state Bajando
    entry: W = -1;
  state Idle
    entry:W = 0;
  state Subiendo_hasta_arriba
    entry: W = 1;
  state Subiendo
    entry: W = 1;
  Subiendo -> Bajand_hasta_abajo [order 4] : [UI==4]
  Bajand_hasta_abajo -> Bajando [order 2] : [UI==3]
  Subiendo -> Bajando [order 3] : [UI==3]
  Bajando -> Bajand_hasta_abajo [order 2] : [UI==4]
  Idle -> Bajando [order 3] : [UI==3&&S>0]
  Subiendo_hasta_arriba -> Bajand_hasta_abajo [order 3] : [UI==4]
  Idle -> Bajand_hasta_abajo [order 4] : [UI==4&&S>0]
  Bajando -> Subiendo [order 3] : [UI==1]
  Subiendo_hasta_arriba -> Bajando [order 4] : [UI==3]
  Bajand_hasta_abajo -> Subiendo [order 4] : [UI==1]
  Bajand_hasta_abajo -> Idle [order 1] : [S<=0]
  Bajand_hasta_abajo -> Subiendo_hasta_arriba [order 3] : [UI==2]
  Bajando -> Idle [order 1] : [S<=0||UI==0]
  Bajando -> Subiendo_hasta_arriba [order 4] : [UI==2]
  (default) -> Idle
  Idle -> Subiendo_hasta_arriba [order 2] : [UI==2&&S<5]
  Idle -> Subiendo [order 1] : [UI == 1&&S<5]
  Subiendo -> Idle [order 1] : [S>=5||UI==0]
  Subiendo_hasta_arriba -> Idle [order 1] : [S >=5]
  Subiendo_hasta_arriba -> Subiendo [order 2] : [UI ==1]
  Subiendo -> Subiendo_hasta_arriba [order 2] : [UI==2]
  data: S input; UI input; W output double

== stateflow chart c00026M_harness/M022/Cyber/WL1/Chart1 ==
  state Bajand_hasta_abajo
    entry: W = -1;
  state Bajando
    entry: W = -1;
  state Idle
    entry:W = 0;
  state Subiendo_hasta_arriba
    entry: W = 1;
  state Subiendo
    entry: W = 1;
  Subiendo -> Bajand_hasta_abajo [order 4] : [UI==4]
  Bajand_hasta_abajo -> Bajando [order 2] : [UI==3]
  Subiendo -> Bajando [order 3] : [UI==3]
  Bajando -> Bajand_hasta_abajo [order 2] : [UI==4]
  Idle -> Bajando [order 3] : [UI==3&&S>0]
  Subiendo_hasta_arriba -> Bajand_hasta_abajo [order 3] : [UI==4]
  Idle -> Bajand_hasta_abajo [order 4] : [UI==4&&S>0]
  Bajando -> Subiendo [order 3] : [UI==1]
  Subiendo_hasta_arriba -> Bajando [order 4] : [UI==3]
  Bajand_hasta_abajo -> Subiendo [order 4] : [UI==1]
  Bajand_hasta_abajo -> Idle [order 1] : [S<=0]
  Bajand_hasta_abajo -> Subiendo_hasta_arriba [order 3] : [UI==2]
  Bajando -> Idle [order 1] : [S<=0||UI==0]
  Bajando -> Subiendo_hasta_arriba [order 4] : [UI==2]
  (default) -> Idle
  Idle -> Subiendo_hasta_arriba [order 2] : [UI==2&&S<5]
  Idle -> Subiendo [order 1] : [UI == 1&&S<5]
  Subiendo -> Idle [order 1] : [S>=5||UI==0]
  Subiendo_hasta_arriba -> Idle [order 1] : [S >=5]
  Subiendo_hasta_arriba -> Subiendo [order 2] : [UI ==1]
  Subiendo -> Subiendo_hasta_arriba [order 2] : [UI==2]
  data: S input; UI input; W output double

== stateflow chart c00026M_harness/M022/Cyber/WL3/Chart2 ==
  state Bajand_hasta_abajo
    entry: W = 0;
  state Bajando
    entry: W = -1;
  state Idle
    entry:W = 0;
  state Subiendo_hasta_arriba
    entry: W = 1;
  state Subiendo
    entry: W = 1;
  Subiendo -> Bajand_hasta_abajo [order 4] : [UI==4]
  Bajand_hasta_abajo -> Bajando [order 2] : [UI==3]
  Subiendo -> Bajando [order 3] : [UI==3]
  Bajando -> Bajand_hasta_abajo [order 2] : [UI==4]
  Idle -> Bajando [order 3] : [UI==3&&S>PosMinW4]
  Subiendo_hasta_arriba -> Bajand_hasta_abajo [order 3] : [UI==4]
  Idle -> Bajand_hasta_abajo [order 4] : [UI==4&&S>PosMinW4]
  Bajando -> Subiendo [order 3] : [UI==1]
  Subiendo_hasta_arriba -> Bajando [order 4] : [UI==3]
  Bajand_hasta_abajo -> Subiendo [order 4] : [UI==1]
  Bajand_hasta_abajo -> Idle [order 1] : [S<=PosMinW4]
  Bajand_hasta_abajo -> Subiendo_hasta_arriba [order 3] : [UI==2]
  Bajando -> Idle [order 1] : [S<=PosMinW4||UI==0]
  Bajando -> Subiendo_hasta_arriba [order 4] : [UI==2]
  (default) -> Idle
  Idle -> Subiendo_hasta_arriba [order 2] : [UI==2&&S<5]
  Idle -> Subiendo [order 1] : [UI == 1&&S<5]
  Subiendo -> Idle [order 1] : [S>=5||UI==0]
  Subiendo_hasta_arriba -> Idle [order 1] : [S >=5]
  Subiendo_hasta_arriba -> Subiendo [order 2] : [UI ==1]
  Subiendo -> Subiendo_hasta_arriba [order 2] : [UI==2]
  data: S input; UI input; W output double; PosMinW4 input

== stateflow chart c00026M_harness/M023/Cyber/WL/Chart ==
  state Bajand_hasta_abajo
    entry: W = -1;
  state Bajando
    entry: W = -1;
  state Idle
    entry:W = 1;
  state Subiendo_hasta_arriba
    entry: W = 1;
  state Subiendo
    entry: W = 1;
  Subiendo -> Bajand_hasta_abajo [order 4] : [UI==4]
  Bajand_hasta_abajo -> Bajando [order 2] : [UI==3]
  Subiendo -> Bajando [order 3] : [UI==3]
  Bajando -> Bajand_hasta_abajo [order 2] : [UI==4]
  Idle -> Bajando [order 3] : [UI==3&&S>0]
  Subiendo_hasta_arriba -> Bajand_hasta_abajo [order 3] : [UI==4]
  Idle -> Bajand_hasta_abajo [order 4] : [UI==4&&S>0]
  Bajando -> Subiendo [order 3] : [UI==1]
  Subiendo_hasta_arriba -> Bajando [order 4] : [UI==3]
  Bajand_hasta_abajo -> Subiendo [order 4] : [UI==1]
  Bajand_hasta_abajo -> Idle [order 1] : [S<=0]
  Bajand_hasta_abajo -> Subiendo_hasta_arriba [order 3] : [UI==2]
  Bajando -> Idle [order 1] : [S<=0||UI==0]
  Bajando -> Subiendo_hasta_arriba [order 4] : [UI==2]
  (default) -> Idle
  Idle -> Subiendo_hasta_arriba [order 2] : [UI==2&&S<5]
  Idle -> Subiendo [order 1] : [UI == 1&&S<5]
  Subiendo -> Idle [order 1] : [S>=5||UI==0]
  Subiendo_hasta_arriba -> Idle [order 1] : [S >=5]
  Subiendo_hasta_arriba -> Subiendo [order 2] : [UI ==1]
  Subiendo -> Subiendo_hasta_arriba [order 2] : [UI==2]
  data: S input; UI input; W output double

== stateflow chart c00026M_harness/M023/Cyber/WL1/Chart1 ==
  state Bajand_hasta_abajo
    entry: W = -1;
  state Bajando
    entry: W = -1;
  state Idle
    entry:W = 0;
  state Subiendo_hasta_arriba
    entry: W = 1;
  state Subiendo
    entry: W = 1;
  Subiendo -> Bajand_hasta_abajo [order 4] : [UI==4]
  Bajand_hasta_abajo -> Bajando [order 2] : [UI==3]
  Subiendo -> Bajando [order 3] : [UI==3]
  Bajando -> Bajand_hasta_abajo [order 2] : [UI==4]
  Idle -> Bajando [order 3] : [UI==3&&S>0]
  Subiendo_hasta_arriba -> Bajand_hasta_abajo [order 3] : [UI==4]
  Idle -> Bajand_hasta_abajo [order 4] : [UI==4&&S>0]
  Bajando -> Subiendo [order 3] : [UI==1]
  Subiendo_hasta_arriba -> Bajando [order 4] : [UI==3]
  Bajand_hasta_abajo -> Subiendo [order 4] : [UI==1]
  Bajand_hasta_abajo -> Idle [order 1] : [S<=0]
  Bajand_hasta_abajo -> Subiendo_hasta_arriba [order 3] : [UI==2]
  Bajando -> Idle [order 1] : [S<=0||UI==0]
  Bajando -> Subiendo_hasta_arriba [order 4] : [UI==2]
  (default) -> Idle
  Idle -> Subiendo_hasta_arriba [order 2] : [UI==2&&S<5]
  Idle -> Subiendo [order 1] : [UI == 1&&S<5]
  Subiendo -> Idle [order 1] : [S>=5||UI==0]
  Subiendo_hasta_arriba -> Idle [order 1] : [S >=5]
  Subiendo_hasta_arriba -> Subiendo [order 2] : [UI ==1]
  Subiendo -> Subiendo_hasta_arriba [order 2] : [UI==2]
  data: S input; UI input; W output double

== stateflow chart c00026M_harness/M023/Cyber/WL3/Chart2 ==
  state Bajand_hasta_abajo
    entry: W = -1;
  state Bajando
    entry: W = -1;
  state Idle
    entry:W = 0;
  state Subiendo_hasta_arriba
    entry: W = 1;
  state Subiendo
    entry: W = 1;
  Subiendo -> Bajand_hasta_abajo [order 4] : [UI==4]
  Bajand_hasta_abajo -> Bajando [order 2] : [UI==3]
  Subiendo -> Bajando [order 3] : [UI==3]
  Bajando -> Bajand_hasta_abajo [order 2] : [UI==4]
  Idle -> Bajando [order 3] : [UI==3&&S>PosMinW4]
  Subiendo_hasta_arriba -> Bajand_hasta_abajo [order 3] : [UI==4]
  Idle -> Bajand_hasta_abajo [order 4] : [UI==4&&S>PosMinW4]
  Bajando -> Subiendo [order 3] : [UI==1]
  Subiendo_hasta_arriba -> Bajando [order 4] : [UI==3]
  Bajand_hasta_abajo -> Subiendo [order 4] : [UI==1]
  Bajand_hasta_abajo -> Idle [order 1] : [S<=PosMinW4]
  Bajand_hasta_abajo -> Subiendo_hasta_arriba [order 3] : [UI==2]
  Bajando -> Idle [order 1] : [S<=PosMinW4||UI==0]
  Bajando -> Subiendo_hasta_arriba [order 4] : [UI==2]
  (default) -> Idle
  Idle -> Subiendo_hasta_arriba [order 2] : [UI==2&&S<5]
  Idle -> Subiendo [order 1] : [UI == 1&&S<5]
  Subiendo -> Idle [order 1] : [S>=5||UI==0]
  Subiendo_hasta_arriba -> Idle [order 1] : [S >=5]
  Subiendo_hasta_arriba -> Subiendo [order 2] : [UI ==1]
  Subiendo -> Subiendo_hasta_arriba [order 2] : [UI==2]
  data: S input; UI input; W output double; PosMinW4 input

== stateflow chart c00026M_harness/M024/Cyber/WL/Chart ==
  state Bajand_hasta_abajo
    entry: W = -1;
  state Bajando
    entry: W = -1;
  state Idle
    entry:W = 0;
  state Subiendo_hasta_arriba
    entry: W = 1;
  state Subiendo
    entry: W = 1;
  Subiendo -> Bajand_hasta_abajo [order 4] : [UI==4]
  Bajand_hasta_abajo -> Bajando [order 2] : [UI==3]
  Subiendo -> Bajando [order 3] : [UI==3]
  Bajando -> Bajand_hasta_abajo [order 2] : [UI==4]
  Idle -> Bajando [order 3] : [UI==3&&S>0]
  Subiendo_hasta_arriba -> Bajand_hasta_abajo [order 3] : [UI==4]
  Idle -> Bajand_hasta_abajo [order 4] : [UI==4&&S>0]
  Bajando -> Subiendo [order 3] : [UI==1]
  Subiendo_hasta_arriba -> Bajando [order 4] : [UI==3]
  Bajand_hasta_abajo -> Subiendo [order 4] : [UI==1]
  Bajand_hasta_abajo -> Idle [order 1] : [S<=0]
  Bajand_hasta_abajo -> Subiendo_hasta_arriba [order 3] : [UI==2]
  Bajando -> Idle [order 1] : [S<=0||UI==0]
  Bajando -> Subiendo_hasta_arriba [order 4] : [UI==2]
  (default) -> Idle
  Idle -> Subiendo_hasta_arriba [order 2] : [UI==2&&S<5]
  Idle -> Subiendo [order 1] : [UI == 1&&S<5]
  Subiendo -> Idle [order 1] : [S>=5||UI==0]
  Subiendo_hasta_arriba -> Idle [order 1] : [S >=5]
  Subiendo_hasta_arriba -> Subiendo [order 2] : [UI ==1]
  Subiendo -> Subiendo_hasta_arriba [order 2] : [UI==2]
  data: S input; UI input; W output double

== stateflow chart c00026M_harness/M024/Cyber/WL1/Chart1 ==
  state Bajand_hasta_abajo
    entry: W = -1;
  state Bajando
    entry: W = -1;
  state Idle
    entry:W = 1;
  state Subiendo_hasta_arriba
    entry: W = 1;
  state Subiendo
    entry: W = 1;
  Subiendo -> Bajand_hasta_abajo [order 4] : [UI==4]
  Bajand_hasta_abajo -> Bajando [order 2] : [UI==3]
  Subiendo -> Bajando [order 3] : [UI==3]
  Bajando -> Bajand_hasta_abajo [order 2] : [UI==4]
  Idle -> Bajando [order 3] : [UI==3&&S>0]
  Subiendo_hasta_arriba -> Bajand_hasta_abajo [order 3] : [UI==4]
  Idle -> Bajand_hasta_abajo [order 4] : [UI==4&&S>0]
  Bajando -> Subiendo [order 3] : [UI==1]
  Subiendo_hasta_arriba -> Bajando [order 4] : [UI==3]
  Bajand_hasta_abajo -> Subiendo [order 4] : [UI==1]
  Bajand_hasta_abajo -> Idle [order 1] : [S<=0]
  Bajand_hasta_abajo -> Subiendo_hasta_arriba [order 3] : [UI==2]
  Bajando -> Idle [order 1] : [S<=0||UI==0]
  Bajando -> Subiendo_hasta_arriba [order 4] : [UI==2]
  (default) -> Idle
  Idle -> Subiendo_hasta_arriba [order 2] : [UI==2&&S<5]
  Idle -> Subiendo [order 1] : [UI == 1&&S<5]
  Subiendo -> Idle [order 1] : [S>=5||UI==0]
  Subiendo_hasta_arriba -> Idle [order 1] : [S >=5]
  Subiendo_hasta_arriba -> Subiendo [order 2] : [UI ==1]
  Subiendo -> Subiendo_hasta_arriba [order 2] : [UI==2]
  data: S input; UI input; W output double

== stateflow chart c00026M_harness/M024/Cyber/WL3/Chart2 ==
  state Bajand_hasta_abajo
    entry: W = -1;
  state Bajando
    entry: W = -1;
  state Idle
    entry:W = 0;
  state Subiendo_hasta_arriba
    entry: W = 1;
  state Subiendo
    entry: W = 1;
  Subiendo -> Bajand_hasta_abajo [order 4] : [UI==4]
  Bajand_hasta_abajo -> Bajando [order 2] : [UI==3]
  Subiendo -> Bajando [order 3] : [UI==3]
  Bajando -> Bajand_hasta_abajo [order 2] : [UI==4]
  Idle -> Bajando [order 3] : [UI==3&&S>PosMinW4]
  Subiendo_hasta_arriba -> Bajand_hasta_abajo [order 3] : [UI==4]
  Idle -> Bajand_hasta_abajo [order 4] : [UI==4&&S>PosMinW4]
  Bajando -> Subiendo [order 3] : [UI==1]
  Subiendo_hasta_arriba -> Bajando [order 4] : [UI==3]
  Bajand_hasta_abajo -> Subiendo [order 4] : [UI==1]
  Bajand_hasta_abajo -> Idle [order 1] : [S<=PosMinW4]
  Bajand_hasta_abajo -> Subiendo_hasta_arriba [order 3] : [UI==2]
  Bajando -> Idle [order 1] : [S<=PosMinW4||UI==0]
  Bajando -> Subiendo_hasta_arriba [order 4] : [UI==2]
  (default) -> Idle
  Idle -> Subiendo_hasta_arriba [order 2] : [UI==2&&S<5]
  Idle -> Subiendo [order 1] : [UI == 1&&S<5]
  Subiendo -> Idle [order 1] : [S>=5||UI==0]
  Subiendo_hasta_arriba -> Idle [order 1] : [S >=5]
  Subiendo_hasta_arriba -> Subiendo [order 2] : [UI ==1]
  Subiendo -> Subiendo_hasta_arriba [order 2] : [UI==2]
  data: S input; UI input; W output double; PosMinW4 input
